simulink library "xbsIO_r2"  (Simulink 5.0)
libraries: xbsIO_r2 x1
settings Model: Creator=administrator  LastModifiedBy=singhj

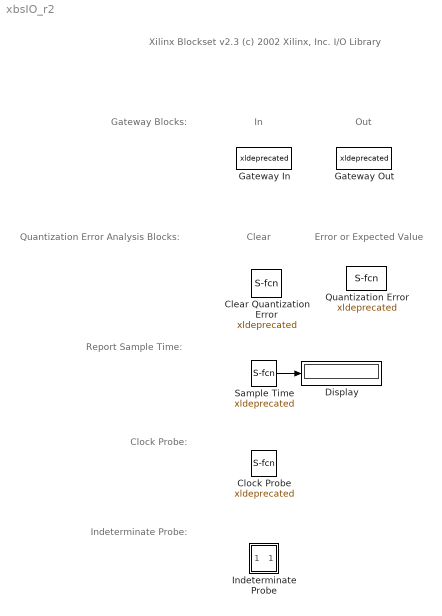
== system xbsIO_r2 ==
  note: Xilinx Blockset v2.3
      | (c) 2002 Xilinx, Inc.
      |
      | I/O Library
  note: Quantization Error Analysis Blocks:
  note: Error or
      | Expected Value
  note: Gateway Blocks:
  note: In
  note: Out
  note: Report Sample Time:
  note: Clear
  note: Clock Probe:
  note: Indeterminate Probe:
  Clear Quantization Error : S-Function  FunctionName=xldeprecated  Parameters=num_inports num_outports  mask(Xilinx Clear Quantization Error Block){opt_port=off}
      mask prompts: opt_port "Add Optional Clear Port"
      mask help:
      | Clear the quantization error tracking mechanism on a trace. Inserting this block has no effect on the computation outside of error analysis sections. Clearing can be controlled through an optional enable port.
      |
      | Hardware notes: In hardware this block costs nothing.
      mask init:
      | [designRoot, family, part, speed, package, simulinkPeriod, sysclkPeriod, dbl_ovrd, trimVbit] = xlSysgenSettings(gcb,0,2);
      | [bg,fg] = xlcmap('XBlock',1);
      | iPos = get_param(gcb,'Position');
      | iWidth=iPos(3)-iPos(1); iHeight=iPos(4)-iPos(2);
      | iCx=iWidth/2;
      | iCy=iHeight/2;
      | if (opt_port==0)
      |   bg = [1 1 1];
      |   shapeX = iCx* (1 + cos(0:pi/6:2*pi));
      |   shapeY = iCy* (1 + sin(0:pi/6:2*pi));
      |   borderX = [];
      |   borderY = [];
      |   bgX = [];
      |   bgY = [];
      |   pnum=1;
      |   pstr='';
      | else
      |   pnum=2;
      |   pstr='*clrE';
      |   shapeX = .8*iCx* (1.25 + cos(0:pi/6:2*pi));
      |   shapeY = .5*iCy* (2.5 + sin(0:pi/6:2*pi));
      |   borderX = [0 0 iWidth iWidth 0 0 iWidth];
      |   borderY = [0 iHeight iHeight 0 0 0.75*iHeight 0.5*iHeight];
      |   bgX=[0 iWidth iWidth 0];  bgY=[0 0 iHeight iHeight];
      | end
      | 
      | % one time added for param list
      | precision0 = 1;
      | has_clr_pin = opt_port;
      | dblOvrd = dbl_ovrd;
      | 
      | % just pass everything to s-function
      | sfcn_mwsv__ = get_param(gcb, 'MaskWSVariables');
      | 
      | num_inports = 1 + opt_port;
      | num_outports = 1;
      | 
      | [bg,fg] = xlcmap('XBlock',1);
      | iPos = get_param(gcb,'Position');
      | iWidth=iPos(3)-iPos(1); iHeight=iPos(4)-iPos(2);
      | iCx=iWidth/2;
      | iCy=iHeight/2;
      | if (opt_port==0)
      |   bg = [1 1 1];
      |   shapeX = iCx* (1 + cos(0:pi/6:2*pi));
      |   shapeY = iCy* (1 + sin(0:pi/6:2*pi));
      |   borderX = [];
      |   borderY = [];
      |   bgX = [];
      |   bgY = [];
      |   pnum=1;
      |   pstr='';
      | else
      |   pnum=2;
      |   pstr='*clrE';
      |   shapeX = .8*iCx* (1.25 + cos(0:pi/6:2*pi));
      |   shapeY = .5*iCy* (2.5 + sin(0:pi/6:2*pi));
      |   borderX = [0 0 iWidth iWidth 0 0 iWidth];
      |   borderY = [0 iHeight iHeight 0 0 0.75*iHeight 0.5*iHeight];
      |   bgX=[0 iWidth iWidth 0];  bgY=[0 0 iHeight iHeight];
      | end
      mask Help: web(xldoclink('Clear Quantization Error'));
      mask Display:
      | patch(bgX,bgY,bg);
      | patch(shapeX,shapeY, [.2 .5 .3]);
      | plot(shapeX,shapeY);
      | plot(borderX, borderY);
      | port_label('input',pnum,pstr);
  Clock Probe : S-Function  FunctionName=xldeprecated  Parameters=-1 -1  mask(Xilinx Clock Probe){}
      mask help:
      | Clock probe.  Produces an output of type double that mirrors the hardware system clock.
      |
      | Hardware notes:  This block is ignored when hardware is generated.
      mask init:
      | [designRoot, family, part, speed, package, simulinkPeriod, sysclkPeriod, dbl_ovrd, trimVbit] = xlSysgenSettings(gcb,0,0);
      | 
      | [bg,fg] = xlcmap('IO');
      | iPos = get_param(gcb,'Position');
      | iWidth=iPos(3)-iPos(1); iHeight=iPos(4)-iPos(2);
      | iCx=iWidth/2;
      | iCy=iHeight/2;
      | shapeX = iCx* (1 + cos(0:pi/6:2*pi));
      | shapeY = iCy* (1 + sin(0:pi/6:2*pi));
      | 
      | % just pass everything to s-function
      | sfcn_mwsv__ = get_param(gcb, 'MaskWSVariables');
      mask Help: web(xldoclink('Clock Probe'));
      mask Display:
      | patch(shapeX,shapeY, bg);
      | plot(shapeX,shapeY);
      | disp('CLK');
  Display : Display
      mask Help: web(xldoclink('Display'));
  Gateway In : S-Function  FunctionName=xldeprecated  Parameters=-1 -1  mask(Xilinx Gateway In){arith_type=Signed  (2's comp), n_bits=8, bin_pt=6, quantization=Truncate, overflow=Wrap, period=1, timing_constraint=None, locs_specified=off, LOCs={}, needs_fixed_name=off, dbl_ovrd=off}
      mask prompts: arith_type "Output Data Type"; n_bits "Number of Bits"; bin_pt "Binary Point"; period "Sample Period"; timing_constraint "IOB Timing Constraint"; locs_specified "Specify IOB Location Constraints"; LOCs "IOB Pad Locations (specify as cell array {'MSB', ..., 'LSB'})"; needs_fixed_name "Do not Prepend Hierarchy to Port Name"; dbl_ovrd "Override with Double"
      mask help:
      | Gateway in block.  Converts inputs of type double to  Xilinx fixed point type.
      |
      | Hardware notes:  In hardware these blocks become top level input ports.
      mask init:
      | [designRoot, family, part, speed, package, simulinkPeriod, sysclkPeriod, dbl_ovrd, trimVbit] = xlSysgenSettings(gcb,1,0);
      | trimVbit = 1;
      | [bg,fg] = xlcmap('IO',dbl_ovrd);
      | iPos = get_param(gcb,'Position');
      | iWidth=iPos(3)-iPos(1); iHeight=iPos(4)-iPos(2);
      | iCx=iWidth/2;
      | iCy=iHeight/2;
      | [logoX, logoY] = xlogo(iPos);
      mask Help: web(xldoclink('Gateway In'));
      mask StyleString: popup(Boolean|Unsigned|Signed  (2's comp)),edit,edit,popup(Truncate|Round  (unbiased: +/- Inf)),popup(Wrap|Saturate|Flag as Error),edit,popup(None|Data Rate|Data Rate;  Set 'FAST' Attribute),checkbox,edit,checkbox,checkbox
      mask Display:
      | patch([0 iWidth iWidth 0],[0 0 iHeight iHeight] , bg);
      | patch(logoX,logoY , fg);
      | port_label('input',1,'dbl');
      | port_label('output',1,'fpt');
      | 
      | ;plot([0 0 iWidth iWidth 0], [0 iHeight iHeight 0 0]);
  Gateway Out : S-Function  FunctionName=xldeprecated  Parameters=-1 -1  mask(Xilinx Gateway Out){hdl_port=on, timing_constraint=None, locs_specified=off, LOCs={}, needs_fixed_name=off}
      mask prompts: hdl_port "Translate into Output Port"; timing_constraint "IOB Timing Constraint"; locs_specified "Specify IOB Location Constraints"; LOCs "IOB Pad Locations (cell array {'MSB', ..., 'LSB'})"; needs_fixed_name "Do not Prepend Hierarchy to Port Name"
      mask help:
      | Gateway out block.  Converts Xilinx fixed point inputs into ouputs of type double.
      |
      | Hardware notes:  In hardware these blocks become top level output ports or are discarded, depending on how they are configured.
      mask init:
      | [designRoot, family, part, speed, package, simulinkPeriod, sysclkPeriod, dbl_ovrd, trimVbit] = xlSysgenSettings(gcb,0,2);
      | [bg,fg] = xlcmap('IO');
      | if (~hdl_port)
      |   [bg,fg]=xlcmap('XBlock',1);
      | end
      | iPos = get_param(gcb,'Position');
      | iWidth=iPos(3)-iPos(1); iHeight=iPos(4)-iPos(2);
      | iCx=iWidth/2;
      | iCy=iHeight/2;
      | [logoX, logoY] = xlogo(iPos);
      mask Help: web(xldoclink('Gateway Out'));
      mask StyleString: checkbox,popup(None|Data Rate|Data Rate;  Set 'FAST' Attribute),checkbox,edit,checkbox
      mask Display:
      | patch([0 iWidth iWidth 0],[0 0 iHeight iHeight] , bg);
      | patch(logoX,logoY , fg);
      | port_label('input',1,'fpt');
      | port_label('output',1,'dbl');
      | 
      | ;plot([0 0 iWidth iWidth 0], [0 iHeight iHeight 0 0]);
  Indeterminate Probe : Subsystem  mask(Xilinx Indeterminate Probe){}
      mask help:
      | Indeterminate Probe.  Produces an output of type double that is 1 when input data is indeterminate.  Output is 0 otherwise.
      |
      | Hardware notes:  This block is ignored when hardware is generated.
      mask init:
      | [designRoot, family, part, speed, package, simulinkPeriod, sysclkPeriod, dbl_ovrd, trimVbit] = xlSysgenSettings(gcb,0,0);
      | 
      | [bg,fg] = xlcmap('IO');
      | iPos = get_param(gcb,'Position');
      | iWidth=iPos(3)-iPos(1); iHeight=iPos(4)-iPos(2);
      | iCx=iWidth/2;
      | iCy=iHeight/2;
      | shapeX = iCx* (1 + cos(0:pi/6:2*pi));
      | shapeY = iCy* (1 + sin(0:pi/6:2*pi));
      mask Help: web(xldoclink('Indeterminate Probe'));
      mask Display:
      | patch(shapeX,shapeY, bg);
      | plot(shapeX,shapeY);
      | disp('!def');
  Quantization Error : S-Function  FunctionName=xldeprecated  Parameters=-1 -1  mask(Xilinx Quantization Error Block){extraction=Quantization Error}
      mask prompts: extraction "Extract"
      mask help:
      | Extracts the quantization error from a Xilinx fixed point signal, or extracts a double value corrected for quantization error. The quantization error is tracked as the difference between the actual value, as represented by the fixed point data, and the expected value, as would be computed under double precision arithmetic.
      |
      | The block can be configured to extract either the quantization error or the expected value (which equals the fixed point value minus the quantization error).
      |
      | Hardware notes:  This block is ignored when hardware is generated.
      mask init:
      | if (extraction==1)
      |   plabel = 'err';
      | else
      |   plabel = 'exp';
      | end
      | 
      | [bg,fg] = xlcmap('IO');
      | iPos = get_param(gcb,'Position');
      | iWidth=iPos(3)-iPos(1); iHeight=iPos(4)-iPos(2);
      | iCx=iWidth/2;
      | iCy=iHeight/2;
      | [logoX, logoY] = xlogo(iPos);
      mask Help: web(xldoclink('Quantization Error'));
      mask StyleString: popup(Quantization Error|Expected Value)
      mask Display:
      | patch([0 iWidth iWidth 0],[0 0 iHeight iHeight] , bg);
      | patch(logoX,logoY , fg);
      | port_label('output',1,plabel);
      | 
      | plot([0 0 iWidth iWidth 0], [0 iHeight iHeight 0 0]);
  Sample Time : S-Function  FunctionName=xldeprecated  Parameters=-1 -1  mask(Xilinx Sample Time Reporter){}
      mask help:
      | Reports the input sample time as an output of type double.
      |
      | Hardware notes: This block is ignored when hardware is generrated.
      mask init:
      | [designRoot, family, part, speed, package, simulinkPeriod, sysclkPeriod, dbl_ovrd, trimVbit] = xlSysgenSettings(gcb,0,0);
      | [bg,fg] = xlcmap('IO');
      | iPos = get_param(gcb,'Position');
      | iWidth=iPos(3)-iPos(1); iHeight=iPos(4)-iPos(2);
      | iCx=iWidth/2;
      | iCy=iHeight/2;
      | shapeX = iCx* (1 + cos(0:pi/6:2*pi));
      | shapeY = iCy* (1 + sin(0:pi/6:2*pi));
      | 
      | 
      | 
      | % one time added for param list
      | 
      | 
      | % just pass everything to s-function
      | sfcn_mwsv__ = get_param(gcb, 'MaskWSVariables');
      mask Help: web(xldoclink('Sample Time'));
      mask Display:
      | patch(shapeX,shapeY, bg);
      | plot(shapeX,shapeY);
      | disp('ST');
  wires:
  Sample Time/1 -> Display/1

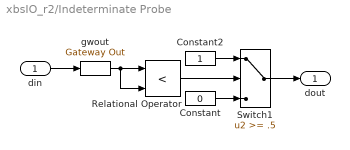
== system xbsIO_r2/Indeterminate Probe ==
  din : Inport
  Constant : Constant  Value=0
  Constant2 : Constant
  Relational Operator : RelationalOperator  Operator=<  InputSameDT=on
  Switch1 : Switch  Threshold=.5  SaturateOnIntegerOverflow=on  InputSameDT=on
  gwout : xbsIO_r2/Gateway Out  hdl_port=off  timing_constraint=None  locs_specified=off  LOCs={}  needs_fixed_name=off
  dout : Outport
  wires:
  din/1 -> gwout/1
  Relational Operator/1 -> Switch1/2
  gwout/1 -> Relational Operator/1, Relational Operator/2
  Constant2/1 -> Switch1/1
  Constant/1 -> Switch1/3
  Switch1/1 -> dout/1
